simulink model "AreaCoverageTestHarness"  (R2016a)
settings: Solver=FixedStepDiscrete  StartTime=0.0  StopTime=16  FixedStep=0.005  RelTol=1e-3
undefined symbols (not defined in the file): EAST, ERRVAL, INIT_COMP_VALUE, INIT_X, INIT_Y, MAX_SPEED, NORTH, PLOT_SAMPLE, ROB_LENG, ROB_WHEEL_R, room, roomSize, SAMPLE_TIME, sigbuilder_block, SOUTH, STEP_SIZE, WEST
(part 1 of 2)
settings Model: Creator=oelkawok  LastModifiedBy=oelkawok

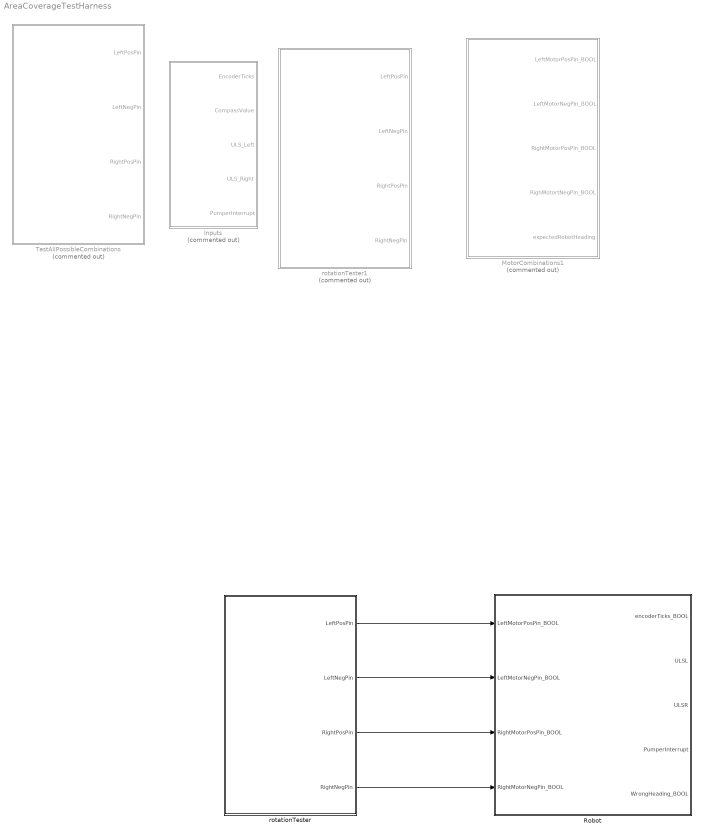
== system AreaCoverageTestHarness ==
  Inputs : Subsystem  Tag=STV Subsys  Commented=on  LoadFcn=sigbuilder_block('load');  StartFcn=sigbuilder_block('start');  StopFcn=sigbuilder_block('stop');  ClipboardFcn=sigbuilder_block('clipboard');  mask(Sigbuilder block){}
      mask help: Simulink:masks:SigbuilderBlock_MD
      mask init:
      | if ~strcmp(get_param(bdroot(gcbh),'SimulationStatus'),'stopped') tuvar = sigbuilder_block('maskInit'); end
      settings: CopyFcn=sigbuilder_block('copy');  DeleteFcn=sigbuilder_block('delete');  ModelCloseFcn=sigbuilder_block('modelClose');  PreSaveFcn=sigbuilder_block('preSave');  PauseFcn=sigbuilder_block('pause');  ContinueFcn=sigbuilder_block('continue');  NameChangeFcn=sigbuilder_block('namechange');  OpenFcn=sigbuilder_block('open',[211.2 103.8 550.8 400.2 ]);  CloseFcn=sigbuilder_block('close');
      mask Display: plot(0, 0, 100, 100,[2, 2, 32, 32, 2], [68, 8, 8, 68, 68],[32, 2], [38, 38], [32, 19, 2],[53, 60, 44], [32, 17, 17, 2],[16, 16, 31, 31]);txt = getActiveGroup(gcbh);text(2, 100, txt,'verticalAlignment', 'top');
  MotorCombinations1 : Subsystem  Commented=on
  Robot : Subsystem
  TestAllPossibleCombinations : Subsystem  Tag=STV Subsys  Commented=on  LoadFcn=sigbuilder_block('load');  StartFcn=sigbuilder_block('start');  StopFcn=sigbuilder_block('stop');  ClipboardFcn=sigbuilder_block('clipboard');  mask(Sigbuilder block){}
      mask help: Simulink:masks:SigbuilderBlock_MD
      mask init:
      | if ~strcmp(get_param(bdroot(gcbh),'SimulationStatus'),'stopped') tuvar = sigbuilder_block('maskInit'); end
      settings: CopyFcn=sigbuilder_block('copy');  DeleteFcn=sigbuilder_block('delete');  ModelCloseFcn=sigbuilder_block('modelClose');  PreSaveFcn=sigbuilder_block('preSave');  PauseFcn=sigbuilder_block('pause');  ContinueFcn=sigbuilder_block('continue');  NameChangeFcn=sigbuilder_block('namechange');  OpenFcn=sigbuilder_block('open',[5.4 28.8 1141.2 525 ]);  CloseFcn=sigbuilder_block('close');
      mask Display: plot(0, 0, 100, 100,[2, 2, 32, 32, 2], [68, 8, 8, 68, 68],[32, 2], [38, 38], [32, 19, 2],[53, 60, 44], [32, 17, 17, 2],[16, 16, 31, 31]);txt = getActiveGroup(gcbh);text(2, 100, txt,'verticalAlignment', 'top');
  rotationTester : Subsystem  Tag=STV Subsys  LoadFcn=sigbuilder_block('load',[6 28.2 1012.8 484.8 ]);  StartFcn=sigbuilder_block('start');  StopFcn=sigbuilder_block('stop');  ClipboardFcn=sigbuilder_block('clipboard');  mask(Sigbuilder block){}
      mask help: Simulink:masks:SigbuilderBlock_MD
      mask init:
      | if ~strcmp(get_param(bdroot(gcbh),'SimulationStatus'),'stopped') tuvar = sigbuilder_block('maskInit'); end
      settings: CopyFcn=sigbuilder_block('copy');  DeleteFcn=sigbuilder_block('delete');  ModelCloseFcn=sigbuilder_block('modelClose');  PreSaveFcn=sigbuilder_block('preSave');  PauseFcn=sigbuilder_block('pause');  ContinueFcn=sigbuilder_block('continue');  NameChangeFcn=sigbuilder_block('namechange');  OpenFcn=sigbuilder_block('open',[5.4 28.8 1141.2 525 ]);  CloseFcn=sigbuilder_block('close');
      mask Display: plot(0, 0, 100, 100,[2, 2, 32, 32, 2], [68, 8, 8, 68, 68],[32, 2], [38, 38], [32, 19, 2],[53, 60, 44], [32, 17, 17, 2],[16, 16, 31, 31]);txt = getActiveGroup(gcbh);text(2, 100, txt,'verticalAlignment', 'top');
  rotationTester1 : Subsystem  Tag=STV Subsys  Commented=on  LoadFcn=sigbuilder_block('load');  StartFcn=sigbuilder_block('start');  StopFcn=sigbuilder_block('stop');  ClipboardFcn=sigbuilder_block('clipboard');  mask(Sigbuilder block){}
      mask help: Simulink:masks:SigbuilderBlock_MD
      mask init:
      | if ~strcmp(get_param(bdroot(gcbh),'SimulationStatus'),'stopped') tuvar = sigbuilder_block('maskInit'); end
      settings: CopyFcn=sigbuilder_block('copy');  DeleteFcn=sigbuilder_block('delete');  ModelCloseFcn=sigbuilder_block('modelClose');  PreSaveFcn=sigbuilder_block('preSave');  PauseFcn=sigbuilder_block('pause');  ContinueFcn=sigbuilder_block('continue');  NameChangeFcn=sigbuilder_block('namechange');  OpenFcn=sigbuilder_block('open',[5.4 28.8 1141.2 525 ]);  CloseFcn=sigbuilder_block('close');
      mask Display: plot(0, 0, 100, 100,[2, 2, 32, 32, 2], [68, 8, 8, 68, 68],[32, 2], [38, 38], [32, 19, 2],[53, 60, 44], [32, 17, 17, 2],[16, 16, 31, 31]);txt = getActiveGroup(gcbh);text(2, 100, txt,'verticalAlignment', 'top');
  wires:
  rotationTester/1(LeftPosPin) -> Robot/1(LeftMotorPosPin_BOOL)
  rotationTester/2(LeftNegPin) -> Robot/2(LeftMotorNegPin_BOOL)
  rotationTester/4(RightNegPin) -> Robot/4(RightMotorNegPin_BOOL)
  rotationTester/3(RightPosPin) -> Robot/3(RightMotorPosPin_BOOL)

== system AreaCoverageTestHarness/Inputs ==
  Demux : Demux  Tag=STV Demux  Outputs=5
  FromWs : FromWorkspace  Tag=STV FromWs  VariableName=tuvar  SampleTime=0
      SigBuilderData=|
      | common.afterFinalStr = 'Extrapolate'
      | common.sampleTime = 0
      | dataSet.timeRange = [0 10]
      | dataSet.name = 'Group 1'
      | sbobj.Groups.Name = 'Group 1'
      | sbobj.Groups.Signals(1).Name = 'EncoderTicks'
      | sbobj.Groups.Signals(1).XData = [0 4 4 6 6 10]
      | sbobj.Groups.Signals(1).YData = [0 0 1 1 0 0]
      | sbobj.Groups.Signals(2).Name = 'CompassValue'
      | sbobj.Groups.Signals(2).XData = [0 4 4 6 6 10]
      | sbobj.Groups.Signals(2).YData = [0 0 1 1 0 0]
      | sbobj.Groups.Signals(3).Name = 'ULS_Left'
      | sbobj.Groups.Signals(3).XData = [0 4 4 6 6 10]
      | sbobj.Groups.Signals(3).YData = [0 0 1 1 0 0]
      | sbobj.Groups.Signals(4).Name = 'ULS_Right'
      | sbobj.Groups.Signals(4).XData = [0 4 4 6 6 10]
      | sbobj.Groups.Signals(4).YData = [0 0 1 1 0 0]
      | sbobj.Groups.Signals(5).Name = 'PumperInterrupt'
      | sbobj.Groups.Signals(5).XData = [0 4 4 6 6 10]
      | sbobj.Groups.Signals(5).YData = [0 0 1 1 0 0]
  EncoderTicks : Outport  Tag=STV Outport
  CompassValue : Outport  Tag=STV Outport  Port=2
  ULS_Left : Outport  Tag=STV Outport  Port=3
  ULS_Right : Outport  Tag=STV Outport  Port=4
  PumperInterrupt : Outport  Tag=STV Outport  Port=5
  wires:
  Demux/1 -> EncoderTicks/1
  FromWs/1 -> Demux/1
  Demux/2 -> CompassValue/1
  Demux/3 -> ULS_Left/1
  Demux/4 -> ULS_Right/1
  Demux/5 -> PumperInterrupt/1

== system AreaCoverageTestHarness/MotorCombinations1 ==
  Signal Builder : Subsystem  Tag=STV Subsys  LoadFcn=sigbuilder_block('load');  StartFcn=sigbuilder_block('start');  StopFcn=sigbuilder_block('stop');  ClipboardFcn=sigbuilder_block('clipboard');  mask(Sigbuilder block){}
      mask help: Simulink:masks:SigbuilderBlock_MD
      mask init:
      | if ~strcmp(get_param(bdroot(gcbh),'SimulationStatus'),'stopped') tuvar = sigbuilder_block('maskInit'); end
      settings: CopyFcn=sigbuilder_block('copy');  DeleteFcn=sigbuilder_block('delete');  ModelCloseFcn=sigbuilder_block('modelClose');  PreSaveFcn=sigbuilder_block('preSave');  PauseFcn=sigbuilder_block('pause');  ContinueFcn=sigbuilder_block('continue');  NameChangeFcn=sigbuilder_block('namechange');  OpenFcn=sigbuilder_block('open',[0 28.8 1152 564 ]);  CloseFcn=sigbuilder_block('close');
      mask Display: plot(0, 0, 100, 100,[2, 2, 32, 32, 2], [68, 8, 8, 68, 68],[32, 2], [38, 38], [32, 19, 2],[53, 60, 44], [32, 17, 17, 2],[16, 16, 31, 31]);txt = getActiveGroup(gcbh);text(2, 100, txt,'verticalAlignment', 'top');
  LeftMotorPosPin_BOOL : Outport
  LeftMotorNegPin_BOOL : Outport  Port=2
  RightMotorPosPin_BOOL : Outport  Port=3
  RighMotortNegPin_BOOL : Outport  Port=4
  expectedRobotHeading : Outport  Port=5
  wires:
  Signal Builder/5(expectedRobotHeading) -> expectedRobotHeading/1
  Signal Builder/1(LeftPosPin) -> LeftMotorPosPin_BOOL/1  "LeftMotorPosPin_BOOL"
  Signal Builder/2(LeftNegPin) -> LeftMotorNegPin_BOOL/1  "LeftMotorNegPin_BOOL"
  Signal Builder/3(RightPosPin) -> RightMotorPosPin_BOOL/1  "RightMotorPosPin_BOOL"
  Signal Builder/4(RightNegPin) -> RighMotortNegPin_BOOL/1  "RighMotortNegPin_BOOL"

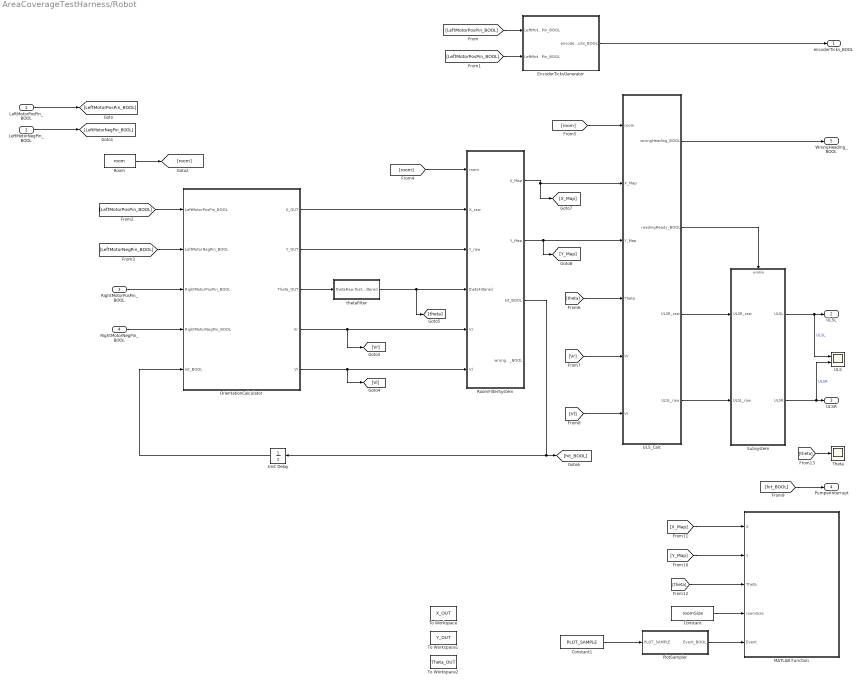
== system AreaCoverageTestHarness/Robot ==
  LeftMotorPosPin_BOOL : Inport
  LeftMotorNegPin_BOOL : Inport  Port=2
  RightMotorPosPin_BOOL : Inport  Port=3
  RightMotorNegPin_BOOL : Inport  Port=4
  Constant : Constant  Value=roomSize
  Constant1 : Constant  Value=PLOT_SAMPLE
  EncoderTicksGenerator : Subsystem
  MATLAB Function : MATLAB Function  TreatAsAtomicUnit=on
  OrientationCalculator : Subsystem
  PlotSampler : Stateflow chart  TreatAsAtomicUnit=on
  Room : Constant  Value=room
  RoomFilterSystem : Subsystem
  Subsystem : Subsystem
  Theta : Scope
  To Workspace : ToWorkspace  VariableName=X_OUT  SaveFormat=Timeseries  SampleTime=-1
  To Workspace1 : ToWorkspace  VariableName=Y_OUT  SaveFormat=Timeseries  SampleTime=-1
  To Workspace2 : ToWorkspace  VariableName=Theta_OUT  SaveFormat=Timeseries  SampleTime=-1
  ULS : Scope  NumInputPorts=2
  ULS_Calc : Subsystem
  Unit Delay : UnitDelay  SampleTime=-1
  thetaFilter : Subsystem
  encoderTicks_BOOL : Outport
  ULSL : Outport  Port=2
  ULSR : Outport  Port=3
  PumperInterrupt : Outport  Port=4
  WrongHeading_BOOL : Outport  Port=5
  wires:
  LeftMotorPosPin_BOOL/1 -> [LeftMotorPosPin_BOOL]
  LeftMotorNegPin_BOOL/1 -> [LeftMotorNegPin_BOOL]
  [LeftMotorPosPin_BOOL] -> EncoderTicksGenerator/2(LeftMotorNegPin_BOOL)
  [LeftMotorPosPin_BOOL] -> EncoderTicksGenerator/1(LeftMotorPosPin_BOOL)
  EncoderTicksGenerator/1(encoderTicks_BOOL) -> encoderTicks_BOOL/1
  [LeftMotorNegPin_BOOL] -> OrientationCalculator/2(LeftMotorNegPin_BOOL)
  [LeftMotorPosPin_BOOL] -> OrientationCalculator/1(LeftMotorPosPin_BOOL)
  RightMotorNegPin_BOOL/1 -> OrientationCalculator/4(RightMotorNegPin_BOOL)
  RightMotorPosPin_BOOL/1 -> OrientationCalculator/3(RightMotorPosPin_BOOL)
  OrientationCalculator/1(X_OUT) -> RoomFilterSystem/2(X_raw)
  OrientationCalculator/2(Y_OUT) -> RoomFilterSystem/3(Y_raw)
  OrientationCalculator/3(Theta_OUT) -> thetaFilter/1(thetaRaw)
  thetaFilter/1(thetaFiltered) -> RoomFilterSystem/4(thetaFiltered), [theta]
  OrientationCalculator/5(Vl) -> [Vl], RoomFilterSystem/6(Vl)
  OrientationCalculator/4(Vr) -> [Vr], RoomFilterSystem/5(Vr)
  RoomFilterSystem/3(hit_BOOL) -> [hit_BOOL], Unit Delay/1
  Unit Delay/1 -> OrientationCalculator/5(hit_BOOL)
  RoomFilterSystem/1(X_Map) -> [X_Map], ULS_Calc/2(X_Map)
  RoomFilterSystem/2(Y_Map) -> [Y_Map], ULS_Calc/3(Y_Map)
  Room/1 -> [room]
  [room] -> RoomFilterSystem/1(room)
  [room] -> ULS_Calc/1(room)
  [theta] -> ULS_Calc/4(Theta)
  [Vr] -> ULS_Calc/5(Vr)
  [Vl] -> ULS_Calc/6(Vl)
  ULS_Calc/2(readingReady_BOOL) -> Subsystem/Enable
  ULS_Calc/4(ULSL_raw) -> Subsystem/2(ULSL_raw)
  ULS_Calc/3(ULSR_raw) -> Subsystem/1(ULSR_raw)
  Subsystem/1(ULSL) -> ULS/1, ULSL/1  "ULSL"
  Subsystem/2(ULSR) -> ULS/2, ULSR/1  "ULSR"
  [hit_BOOL] -> PumperInterrupt/1
  ULS_Calc/1(wrongHeading_BOOL) -> WrongHeading_BOOL/1
  [theta] -> Theta/1
  [Y_Map] -> MATLAB Function/2(Y)
  [X_Map] -> MATLAB Function/1(X)
  [theta] -> MATLAB Function/3(Theta)
  Constant/1 -> MATLAB Function/4(roomSize)
  PlotSampler/1(Event_BOOL) -> MATLAB Function/5(Event)
  Constant1/1 -> PlotSampler/1(PLOT_SAMPLE)

== system AreaCoverageTestHarness/TestAllPossibleCombinations ==
  Demux : Demux  Tag=STV Demux
  FromWs : FromWorkspace  Tag=STV FromWs  VariableName=tuvar  SampleTime=0
      SigBuilderData=|
      | common.afterFinalStr = 'Extrapolate'
      | common.sampleTime = 0
      | dataSet.timeRange = [0 16]
      | dataSet.name = 'Group 1'
      | sbobj.Groups.Name = 'Group 1'
      | sbobj.Groups.Signals(1).Name = 'LeftPosPin'
      | sbobj.Groups.Signals(1).XData = [0 8 8 13.8 16]
      | sbobj.Groups.Signals(1).YData = [0 0 1 1 1]
      | sbobj.Groups.Signals(2).Name = 'LeftNegPin'
      | sbobj.Groups.Signals(2).XData = [0 1 2 4 4 8 8 12 12 16]
      | sbobj.Groups.Signals(2).YData = [0 0 0 0 1 1 0 0 1 1]
      | sbobj.Groups.Signals(3).Name = 'RightPosPin'
      | sbobj.Groups.Signals(3).XData = [0 1 2 4 4 6 8 8 10 10 12 12 14 14 16]
      | sbobj.Groups.Signals(3).YData = [0 0 0 0 1 1 1 0 0 1 1 0 0 1 1]
      | sbobj.Groups.Signals(4).Name = 'RightNegPin'
      | sbobj.Groups.Signals(4).XData = [0 1 1 3.08 3.08 8 11 11 12 12 13 13 14 14 15 15 16]
      | sbobj.Groups.Signals(4).YData = [0 0 1 1 0 0 0 1 1 0 0 1 1 0 0 1 1]
      | sbobj.Groups.TimeRange = [0 16]
  LeftPosPin : Outport  Tag=STV Outport
  LeftNegPin : Outport  Tag=STV Outport  Port=2
  RightPosPin : Outport  Tag=STV Outport  Port=3
  RightNegPin : Outport  Tag=STV Outport  Port=4
  wires:
  Demux/1 -> LeftPosPin/1
  FromWs/1 -> Demux/1
  Demux/2 -> LeftNegPin/1
  Demux/3 -> RightPosPin/1
  Demux/4 -> RightNegPin/1

== system AreaCoverageTestHarness/rotationTester ==
  Demux : Demux  Tag=STV Demux
  FromWs : FromWorkspace  Tag=STV FromWs  VariableName=tuvar  SampleTime=0
      SigBuilderData=|
      | common.afterFinalStr = 'Extrapolate'
      | common.sampleTime = 0
      | dataSet.timeRange = [0 16]
      | dataSet.name = 'Group 1'
      | sbobj.Groups.Name = 'Group 1'
      | sbobj.Groups.Signals(1).Name = 'LeftPosPin'
      | sbobj.Groups.Signals(1).XData = [0 2 3.35 8 8 12.16 12.16 16]
      | sbobj.Groups.Signals(1).YData = [1 1 1 1 0 0 1 1]
      | sbobj.Groups.Signals(2).Name = 'LeftNegPin'
      | sbobj.Groups.Signals(2).XData = [0 1 2.18 10 10 12 12 16]
      | sbobj.Groups.Signals(2).YData = [0 0 0 0 1 1 0 0]
      | sbobj.Groups.Signals(3).Name = 'RightPosPin'
      | sbobj.Groups.Signals(3).XData = [0 1 2 8 12.28 12.28 16]
      | sbobj.Groups.Signals(3).YData = [0 0 0 0 0 1 1]
      | sbobj.Groups.Signals(4).Name = 'RightNegPin'
      | sbobj.Groups.Signals(4).XData = [0 2 3.35 8 8 10 10 12 12 16]
      | sbobj.Groups.Signals(4).YData = [1 1 1 1 0 0 1 1 0 0]
      | sbobj.Groups.TimeRange = [0 16]
  LeftPosPin : Outport  Tag=STV Outport
  LeftNegPin : Outport  Tag=STV Outport  Port=2
  RightPosPin : Outport  Tag=STV Outport  Port=3
  RightNegPin : Outport  Tag=STV Outport  Port=4
  wires:
  Demux/4 -> RightNegPin/1
  Demux/3 -> RightPosPin/1
  Demux/2 -> LeftNegPin/1
  FromWs/1 -> Demux/1
  Demux/1 -> LeftPosPin/1

== system AreaCoverageTestHarness/rotationTester1 ==
  Demux : Demux  Tag=STV Demux
  FromWs : FromWorkspace  Tag=STV FromWs  VariableName=tuvar  SampleTime=0
      SigBuilderData=|
      | common.afterFinalStr = 'Extrapolate'
      | common.sampleTime = 0
      | dataSet.timeRange = [0 16]
      | dataSet.name = 'Group 1'
      | sbobj.Groups.Name = 'Group 1'
      | sbobj.Groups.Signals(1).Name = 'LeftPosPin'
      | sbobj.Groups.Signals(1).XData = [0 2.14 2.14 13.8 16]
      | sbobj.Groups.Signals(1).YData = [0 0 1 1 1]
      | sbobj.Groups.Signals(2).Name = 'LeftNegPin'
      | sbobj.Groups.Signals(2).XData = [0 1 1 2.08 2.08 12 16]
      | sbobj.Groups.Signals(2).YData = [0 0 1 1 0 0 0]
      | sbobj.Groups.Signals(3).Name = 'RightPosPin'
      | sbobj.Groups.Signals(3).XData = [0 1 2.08 2.08 13.18 14 14 16]
      | sbobj.Groups.Signals(3).YData = [0 0 0 1 1 1 0 0]
      | sbobj.Groups.Signals(4).Name = 'RightNegPin'
      | sbobj.Groups.Signals(4).XData = [0 1 1 8 11 12 13 14 15 16]
      | sbobj.Groups.Signals(4).YData = [0 0 1 1 1 1 1 1 1 1]
      | sbobj.Groups.TimeRange = [0 16]
  LeftPosPin : Outport  Tag=STV Outport
  LeftNegPin : Outport  Tag=STV Outport  Port=2
  RightPosPin : Outport  Tag=STV Outport  Port=3
  RightNegPin : Outport  Tag=STV Outport  Port=4
  wires:
  Demux/1 -> LeftPosPin/1
  FromWs/1 -> Demux/1
  Demux/2 -> LeftNegPin/1
  Demux/3 -> RightPosPin/1
  Demux/4 -> RightNegPin/1

== system AreaCoverageTestHarness/MotorCombinations1/Signal Builder ==
  Demux : Demux  Tag=STV Demux  Outputs=5
  FromWs : FromWorkspace  Tag=STV FromWs  VariableName=tuvar  SampleTime=0
      SigBuilderData=|
      | common.afterFinalStr = 'Extrapolate'
      | common.sampleTime = 0
      | dataSet.timeRange = [0 16]
      | dataSet.name = 'Group 1'
      | sbobj.Groups.Name = 'Group 1'
      | sbobj.Groups.Signals(1).Name = 'LeftPosPin'
      | sbobj.Groups.Signals(1).XData = [0 8 8 13.8 16]
      | sbobj.Groups.Signals(1).YData = [0 0 1 1 1]
      | sbobj.Groups.Signals(2).Name = 'LeftNegPin'
      | sbobj.Groups.Signals(2).XData = [0 1 2 4 4 8 8 12 12 16]
      | sbobj.Groups.Signals(2).YData = [0 0 0 0 1 1 0 0 1 1]
      | sbobj.Groups.Signals(3).Name = 'RightPosPin'
      | sbobj.Groups.Signals(3).XData = [0 1 2 2 4 4 6 6 8 8 10 10 12 12 14 14 16]
      | sbobj.Groups.Signals(3).YData = [0 0 0 1 1 0 0 1 1 0 0 1 1 0 0 1 1]
      | sbobj.Groups.Signals(4).Name = 'RightNegPin'
      | sbobj.Groups.Signals(4).XData = [0 1 1 2 2 3 3 4 4 5 5 6 6 7 7 8 8 9 9 10 10 11 11 12 12 13 13 14 14 15 15 16]
      | sbobj.Groups.Signals(4).YData = [0 0 1 1 0 0 1 1 0 0 1 1 0 0 1 1 0 0 1 1 0 0 1 1 0 0 1 1 0 0 1 1]
      | sbobj.Groups.Signals(5).Name = 'expectedRobotHeading'
      | sbobj.Groups.Signals(5).XData = [0 1 1 2 2 3 3 4 4 5 5 6 6 7 7 8 8 9 9 10 10 11 11 12 12 13 13 14 14 15 15 16]
      | sbobj.Groups.Signals(5).YData = [7 7 2 2 1 1 7 7 1 1 6 6 3 3 1 1 2 2 4 4 5 5 2 2 7 7 2 2 1 1 7 7]
      | sbobj.Groups.TimeRange = [0 16]
  LeftPosPin : Outport  Tag=STV Outport
  LeftNegPin : Outport  Tag=STV Outport  Port=2
  RightPosPin : Outport  Tag=STV Outport  Port=3
  RightNegPin : Outport  Tag=STV Outport  Port=4
  expectedRobotHeading : Outport  Tag=STV Outport  Port=5
  wires:
  Demux/5 -> expectedRobotHeading/1
  Demux/4 -> RightNegPin/1
  Demux/3 -> RightPosPin/1
  Demux/2 -> LeftNegPin/1
  FromWs/1 -> Demux/1
  Demux/1 -> LeftPosPin/1

== system AreaCoverageTestHarness/Robot/EncoderTicksGenerator ==
  LeftMotorPosPin_BOOL : Inport
  LeftMotorNegPin_BOOL : Inport  Port=2
  Logical Operator : Logic  Operator=XOR  AllPortsSameDT=off  OutDataTypeStr=boolean
  SquareWaveCreatorLeft : Stateflow chart  TreatAsAtomicUnit=on
  encoderTicks_BOOL : Outport
  wires:
  LeftMotorNegPin_BOOL/1 -> Logical Operator/2
  LeftMotorPosPin_BOOL/1 -> Logical Operator/1
  Logical Operator/1 -> SquareWaveCreatorLeft/1(ControlSignal_BOOL_in)
  SquareWaveCreatorLeft/1(encoderTicks_BOOL) -> encoderTicks_BOOL/1

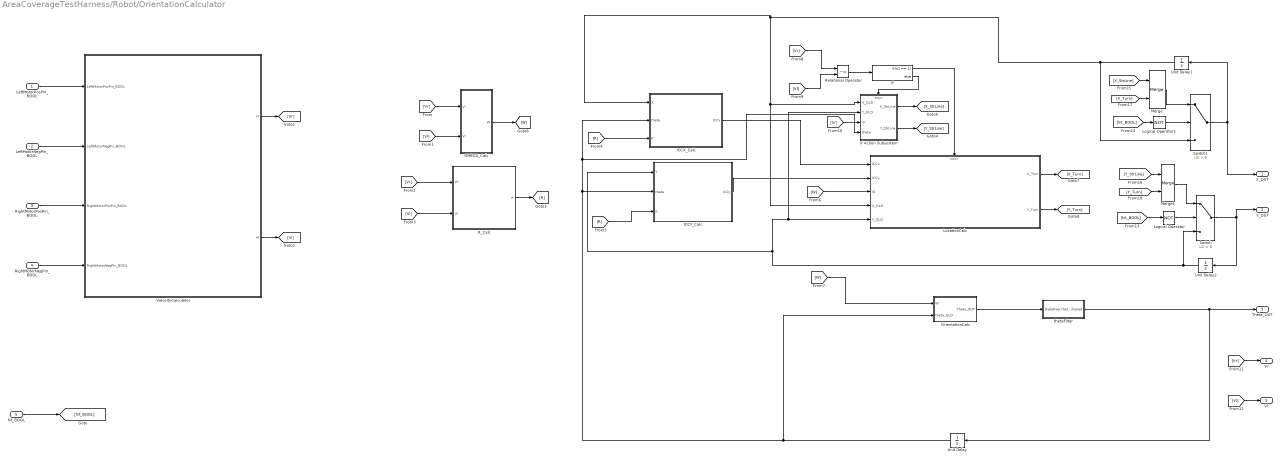
== system AreaCoverageTestHarness/Robot/OrientationCalculator ==
  LeftMotorPosPin_BOOL : Inport
  LeftMotorNegPin_BOOL : Inport  Port=2
  RightMotorPosPin_BOOL : Inport  Port=3
  RightMotorNegPin_BOOL : Inport  Port=4
  hit_BOOL : Inport  Port=5
  ICCX_Calc : Subsystem
  ICCY_Calc : Subsystem
  If : If  IfExpression=u1 == 1
  If Action Subsystem : Subsystem  TreatAsAtomicUnit=on
  LocationCalc : Subsystem
  Logical Operator : Logic  Operator=NOT  AllPortsSameDT=off  OutDataTypeStr=boolean
  Logical Operator1 : Logic  Operator=NOT  AllPortsSameDT=off  OutDataTypeStr=boolean
  Merge : Merge
  Merge1 : Merge
  OMEGA_Calc : Subsystem
  OrientationCalc : Subsystem
  R_Calc : Subsystem
  Relational Operator : RelationalOperator  Operator=~=  OutDataTypeStr=boolean
  Switch : Switch  Criteria=u2 > Threshold
  Switch1 : Switch  Criteria=u2 > Threshold
  Unit Delay : UnitDelay  InitialCondition=INIT_COMP_VALUE  SampleTime=-1
  Unit Delay1 : UnitDelay  InitialCondition=INIT_X  SampleTime=-1
  Unit Delay2 : UnitDelay  InitialCondition=INIT_Y  SampleTime=-1
  VelocityCalculator : Subsystem
  thetaFilter : Subsystem
  X_OUT : Outport
  Y_OUT : Outport  Port=2
  Theta_OUT : Outport  Port=3
  Vr : Outport  Port=4
  Vl : Outport  Port=5
  wires:
  [Vr] -> OMEGA_Calc/1(Vr)
  [Vl] -> OMEGA_Calc/2(Vl)
  [Vr] -> R_Calc/1(Vr)
  [Vl] -> R_Calc/2(Vl)
  R_Calc/1(R) -> [R]
  Unit Delay1/1 -> ICCX_Calc/1(X), If Action Subsystem/1(X_OLD), LocationCalc/4(X_OLD), Switch1/3
  Unit Delay/1 -> OrientationCalc/2(theta_OLD), ICCY_Calc/2(theta), If Action Subsystem/4(theta), ICCX_Calc/2(theta)
  [R] -> ICCX_Calc/3(R)
  Unit Delay2/1 -> Switch/3, ICCY_Calc/1(Y), If Action Subsystem/2(Y_OLD), LocationCalc/5(Y_OLD)
  [R] -> ICCY_Calc/3(R)
  ICCX_Calc/1(ICCx) -> LocationCalc/1(ICCx)
  ICCY_Calc/1(ICCy) -> LocationCalc/2(ICCy)
  OMEGA_Calc/1(W) -> [W]
  Merge1/1 -> Switch/1
  [W] -> LocationCalc/3(W)
  OrientationCalc/1(Theta_OUT) -> thetaFilter/1(thetaRaw)
  [W] -> OrientationCalc/1(W)
  [Vl] -> Relational Operator/2
  [Vr] -> Relational Operator/1
  Relational Operator/1 -> If/1
  If/1 -> LocationCalc/Action
  If/2 -> If Action Subsystem/Action
  [Vr] -> If Action Subsystem/3(Vr)
  thetaFilter/1(thetaFiltered) -> Unit Delay/1, Theta_OUT/1
  [Vl] -> Vl/1
  [Vr] -> Vr/1
  hit_BOOL/1 -> [hit_BOOL]
  [hit_BOOL] -> Logical Operator/1
  Logical Operator/1 -> Switch/2
  Switch/1 -> Unit Delay2/1, Y_OUT/1
  [hit_BOOL] -> Logical Operator1/1
  Logical Operator1/1 -> Switch1/2
  Merge/1 -> Switch1/1
  Switch1/1 -> Unit Delay1/1, X_OUT/1
  LeftMotorPosPin_BOOL/1 -> VelocityCalculator/1(LeftMotorPosPin_BOOL)
  LeftMotorNegPin_BOOL/1 -> VelocityCalculator/2(LeftMotorNegPin_BOOL)
  RightMotorPosPin_BOOL/1 -> VelocityCalculator/3(RightMotorPosPin_BOOL)
  RightMotorNegPin_BOOL/1 -> VelocityCalculator/4(RightMotorNegPin_BOOL)
  VelocityCalculator/1(Vr) -> [Vr]
  VelocityCalculator/2(Vl) -> [Vl]
  [X_StrLine] -> Merge/1
  If Action Subsystem/1(X_StrLine) -> [X_StrLine]
  If Action Subsystem/2(Y_StrLine) -> [Y_StrLine]
  [Y_StrLine] -> Merge1/1
  LocationCalc/1(X_Turn) -> [X_Turn]
  [X_Turn] -> Merge/2
  LocationCalc/2(Y_Turn) -> [Y_Turn]
  [Y_Turn] -> Merge1/2

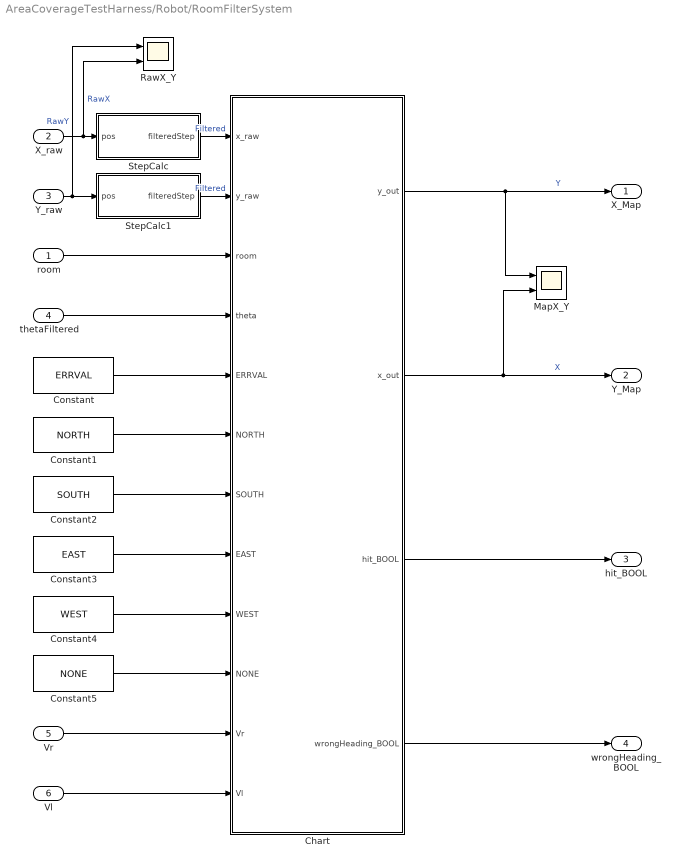
== system AreaCoverageTestHarness/Robot/RoomFilterSystem ==
  room : Inport
  X_raw : Inport  Port=2
  Y_raw : Inport  Port=3
  thetaFiltered : Inport  Port=4
  Vr : Inport  Port=5
  Vl : Inport  Port=6
  Chart : Stateflow chart  TreatAsAtomicUnit=on
  Constant : Constant  Value=ERRVAL
  Constant1 : Constant  Value=NORTH
  Constant2 : Constant  Value=SOUTH
  Constant3 : Constant  Value=EAST
  Constant4 : Constant  Value=WEST
  Constant5 : Constant  Value=NONE
  MapX_Y : Scope  NumInputPorts=2
  RawX_Y : Scope  NumInputPorts=2
  StepCalc : Subsystem
  StepCalc1 : Subsystem
  X_Map : Outport
  Y_Map : Outport  Port=2
  hit_BOOL : Outport  Port=3
  wrongHeading_BOOL : Outport  Port=4
  wires:
  Y_raw/1 -> RawX_Y/1, StepCalc1/1(pos)  "RawY"
  room/1 -> Chart/3(room)
  Chart/1(y_out) -> MapX_Y/1, X_Map/1  "Y"
  Chart/2(x_out) -> MapX_Y/2, Y_Map/1  "X"
  thetaFiltered/1 -> Chart/4(theta)
  Constant/1 -> Chart/5(ERRVAL)
  Constant1/1 -> Chart/6(NORTH)
  Constant2/1 -> Chart/7(SOUTH)
  Constant5/1 -> Chart/10(NONE)
  Constant4/1 -> Chart/9(WEST)
  Constant3/1 -> Chart/8(EAST)
  Vr/1 -> Chart/11(Vr)
  Vl/1 -> Chart/12(Vl)
  Chart/3(hit_BOOL) -> hit_BOOL/1
  Chart/4(wrongHeading_BOOL) -> wrongHeading_BOOL/1
  StepCalc1/1(filteredStep) -> Chart/2(y_raw)  "Filtered"
  X_raw/1 -> RawX_Y/2, StepCalc/1(pos)  "RawX"
  StepCalc/1(filteredStep) -> Chart/1(x_raw)  "Filtered"

== system AreaCoverageTestHarness/Robot/Subsystem ==
  ULSR_raw : Inport
  ULSL_raw : Inport  Port=2
  Enable : EnablePort
  ULSL : Outport
  ULSR : Outport  Port=2
  wires:
  ULSL_raw/1 -> ULSR/1
  ULSR_raw/1 -> ULSL/1

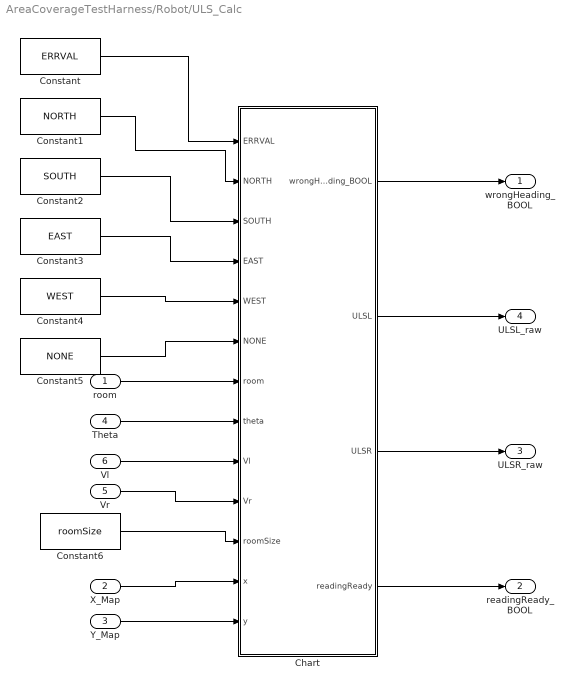
== system AreaCoverageTestHarness/Robot/ULS_Calc ==
  room : Inport
  X_Map : Inport  Port=2
  Y_Map : Inport  Port=3
  Theta : Inport  Port=4
  Vr : Inport  Port=5
  Vl : Inport  Port=6
  Chart : Stateflow chart  TreatAsAtomicUnit=on
  Constant : Constant  Value=ERRVAL
  Constant1 : Constant  Value=NORTH
  Constant2 : Constant  Value=SOUTH
  Constant3 : Constant  Value=EAST
  Constant4 : Constant  Value=WEST
  Constant5 : Constant  Value=NONE
  Constant6 : Constant  Value=roomSize
  wrongHeading_BOOL : Outport
  readingReady_BOOL : Outport  Port=2
  ULSR_raw : Outport  Port=3
  ULSL_raw : Outport  Port=4
  wires:
  X_Map/1 -> Chart/12(x)
  Y_Map/1 -> Chart/13(y)
  Theta/1 -> Chart/8(theta)
  Constant4/1 -> Chart/5(WEST)
  Constant5/1 -> Chart/6(NONE)
  Constant3/1 -> Chart/4(EAST)
  Constant2/1 -> Chart/3(SOUTH)
  Constant1/1 -> Chart/2(NORTH)
  Constant/1 -> Chart/1(ERRVAL)
  room/1 -> Chart/7(room)
  Constant6/1 -> Chart/11(roomSize)
  Vl/1 -> Chart/9(Vl)
  Vr/1 -> Chart/10(Vr)
  Chart/2(ULSL) -> ULSL_raw/1
  Chart/3(ULSR) -> ULSR_raw/1
  Chart/4(readingReady) -> readingReady_BOOL/1
  Chart/1(wrongHeading_BOOL) -> wrongHeading_BOOL/1

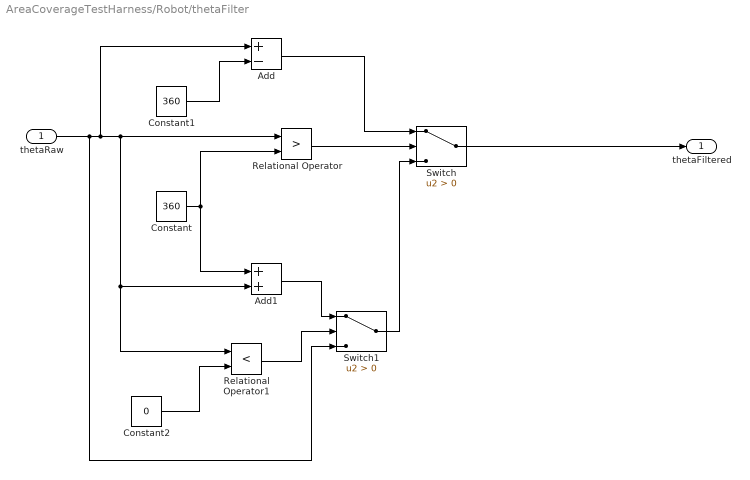
== system AreaCoverageTestHarness/Robot/thetaFilter ==
  thetaRaw : Inport
  Add : Sum  Inputs=+-
  Add1 : Sum
  Constant : Constant  Value=360
  Constant1 : Constant  Value=360
  Constant2 : Constant  Value=0
  Relational Operator : RelationalOperator  Operator=>  OutDataTypeStr=boolean
  Relational Operator1 : RelationalOperator  Operator=<  OutDataTypeStr=boolean
  Switch : Switch  Criteria=u2 > Threshold
  Switch1 : Switch  Criteria=u2 > Threshold
  thetaFiltered : Outport
  wires:
  thetaRaw/1 -> Switch1/3, Add/1, Add1/2, Relational Operator1/1, Relational Operator/1
  Constant/1 -> Add1/1, Relational Operator/2
  Relational Operator/1 -> Switch/2
  Constant1/1 -> Add/2
  Add/1 -> Switch/1
  Constant2/1 -> Relational Operator1/2
  Relational Operator1/1 -> Switch1/2
  Add1/1 -> Switch1/1
  Switch1/1 -> Switch/3
  Switch/1 -> thetaFiltered/1

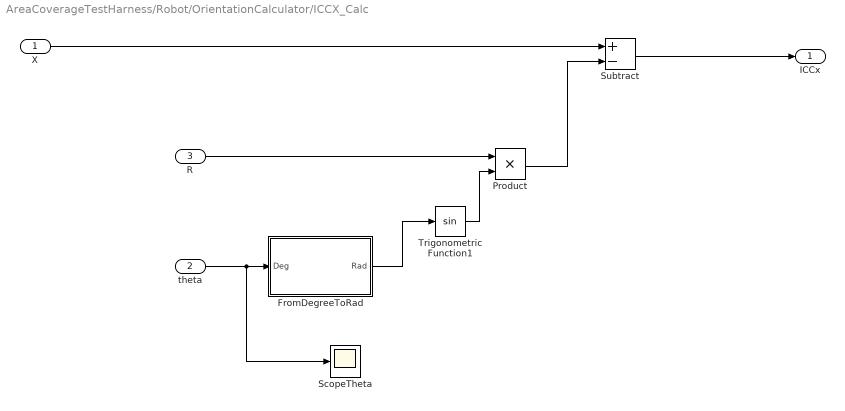
== system AreaCoverageTestHarness/Robot/OrientationCalculator/ICCX_Calc ==
  X : Inport
  theta : Inport  Port=2
  R : Inport  Port=3
  FromDegreeToRad : Subsystem
  Product : Product
  ScopeTheta : Scope
  Subtract : Sum  Inputs=+-
  Trigonometric Function1 : Trigonometry
  ICCx : Outport
  wires:
  Product/1 -> Subtract/2
  X/1 -> Subtract/1
  FromDegreeToRad/1(Rad) -> Trigonometric Function1/1
  Subtract/1 -> ICCx/1
  theta/1 -> ScopeTheta/1, FromDegreeToRad/1(Deg)
  Trigonometric Function1/1 -> Product/2
  R/1 -> Product/1

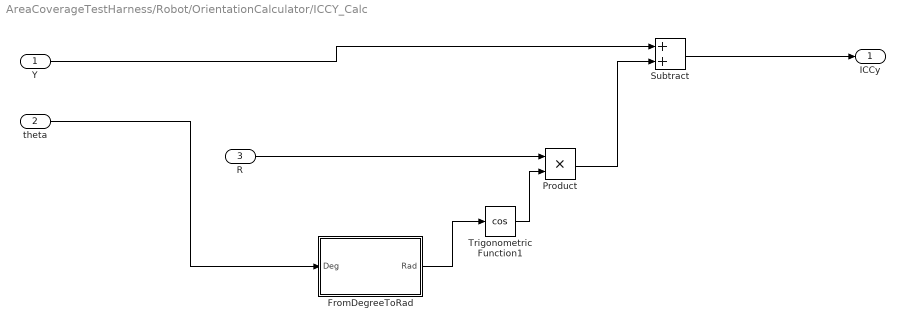
== system AreaCoverageTestHarness/Robot/OrientationCalculator/ICCY_Calc ==
  Y : Inport
  theta : Inport  Port=2
  R : Inport  Port=3
  FromDegreeToRad : Subsystem
  Product : Product
  Subtract : Sum
  Trigonometric Function1 : Trigonometry  Operator=cos
  ICCy : Outport
  wires:
  Y/1 -> Subtract/1
  Trigonometric Function1/1 -> Product/2
  theta/1 -> FromDegreeToRad/1(Deg)
  Subtract/1 -> ICCy/1
  FromDegreeToRad/1(Rad) -> Trigonometric Function1/1
  Product/1 -> Subtract/2
  R/1 -> Product/1

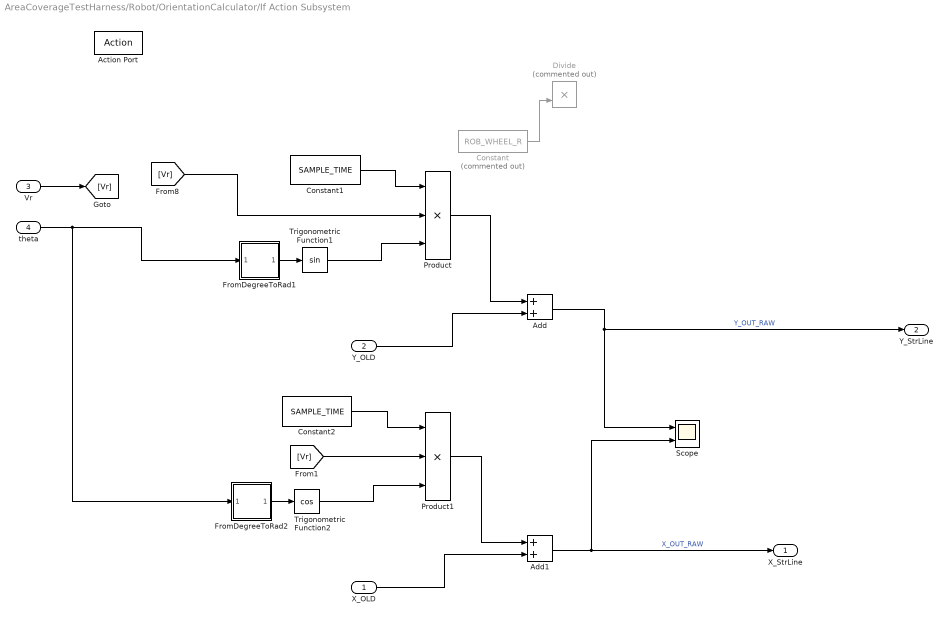
== system AreaCoverageTestHarness/Robot/OrientationCalculator/If Action Subsystem ==
  X_OLD : Inport
  Y_OLD : Inport  Port=2
  Vr : Inport  Port=3
  theta : Inport  Port=4
  Action Port : ActionPort  ActionType=else
  Add : Sum
  Add1 : Sum
  Constant : Constant  Commented=on  Value=ROB_WHEEL_R
  Constant1 : Constant  Value=SAMPLE_TIME  SampleTime=-1
  Constant2 : Constant  Value=SAMPLE_TIME  SampleTime=-1
  Divide : Product  Commented=on  Inputs=**
  FromDegreeToRad1 : Subsystem
  FromDegreeToRad2 : Subsystem
  Product : Product  Inputs=3
  Product1 : Product  Inputs=3
  Scope : Scope  NumInputPorts=2
  Trigonometric Function1 : Trigonometry
  Trigonometric Function2 : Trigonometry  Operator=cos
  X_StrLine : Outport
  Y_StrLine : Outport  Port=2
  wires:
  FromDegreeToRad1/1(Rad) -> Trigonometric Function1/1
  Trigonometric Function1/1 -> Product/3
  Vr/1 -> [Vr]
  theta/1 -> FromDegreeToRad2/1(Deg), FromDegreeToRad1/1(Deg)
  Constant1/1 -> Product/1
  Y_OLD/1 -> Add/2
  Product/1 -> Add/1
  Add/1 -> Y_StrLine/1, Scope/1  "Y_OUT_RAW"
  FromDegreeToRad2/1(Rad) -> Trigonometric Function2/1
  Trigonometric Function2/1 -> Product1/3
  [Vr] -> Product1/2
  Constant2/1 -> Product1/1
  X_OLD/1 -> Add1/2
  Product1/1 -> Add1/1
  Add1/1 -> Scope/2, X_StrLine/1  "X_OUT_RAW"
  [Vr] -> Product/2
  Constant/1 -> Divide/2

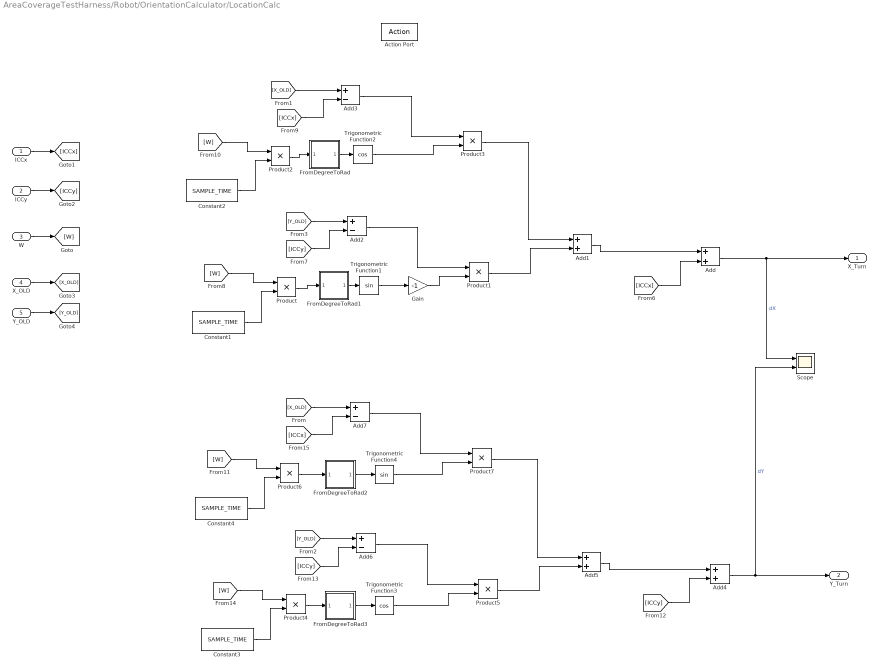
== system AreaCoverageTestHarness/Robot/OrientationCalculator/LocationCalc ==
  ICCx : Inport
  ICCy : Inport  Port=2
  W : Inport  Port=3
  X_OLD : Inport  Port=4
  Y_OLD : Inport  Port=5
  Action Port : ActionPort  ActionType=then
  Add{,1,4..5} (4 alike) : Sum
  Add{2..3,6..7} (4 alike) : Sum  Inputs=+-
  Constant{1..4} (4 alike) : Constant  Value=SAMPLE_TIME  SampleTime=-1
  FromDegreeToRad : Subsystem
  FromDegreeToRad1 : Subsystem
  FromDegreeToRad2 : Subsystem
  FromDegreeToRad3 : Subsystem
  Gain : Gain  Gain=-1
  Product{,1..7} (8 alike) : Product
  Scope : Scope  NumInputPorts=2
  Trigonometric Function1 : Trigonometry
  Trigonometric Function2 : Trigonometry  Operator=cos
  Trigonometric Function3 : Trigonometry  Operator=cos
  Trigonometric Function4 : Trigonometry
  X_Turn : Outport
  Y_Turn : Outport  Port=2
  wires:
  [W] -> Product/1
  Gain/1 -> Product1/2
  [ICCx] -> Add/2
  Add2/1 -> Product1/1
  Add1/1 -> Add/1
  Product2/1 -> FromDegreeToRad/1(Deg)
  Product1/1 -> Add1/2
  Constant1/1 -> Product/2
  Add3/1 -> Product3/1
  Add/1 -> Scope/1, X_Turn/1  "dX"
  Product/1 -> FromDegreeToRad1/1(Deg)
  Trigonometric Function1/1 -> Gain/1
  [ICCy] -> Add2/2
  Constant2/1 -> Product2/2
  Trigonometric Function2/1 -> Product3/2
  [ICCx] -> Add3/2
  [W] -> Product2/1
  Product3/1 -> Add1/1
  Add6/1 -> Product5/1
  [ICCy] -> Add4/2
  Product5/1 -> Add5/2
  Product7/1 -> Add5/1
  Add7/1 -> Product7/1
  Product6/1 -> FromDegreeToRad2/1(Deg)
  Trigonometric Function3/1 -> Product5/2
  Add5/1 -> Add4/1
  Trigonometric Function4/1 -> Product7/2
  [W] -> Product4/1
  Add4/1 -> Scope/2, Y_Turn/1  "dY"
  [ICCy] -> Add6/2
  [ICCx] -> Add7/2
  Constant3/1 -> Product4/2
  Product4/1 -> FromDegreeToRad3/1(Deg)
  [W] -> Product6/1
  Constant4/1 -> Product6/2
  W/1 -> [W]
  ICCx/1 -> [ICCx]
  ICCy/1 -> [ICCy]
  FromDegreeToRad/1(Rad) -> Trigonometric Function2/1
  FromDegreeToRad1/1(Rad) -> Trigonometric Function1/1
  FromDegreeToRad2/1(Rad) -> Trigonometric Function4/1
  FromDegreeToRad3/1(Rad) -> Trigonometric Function3/1
  X_OLD/1 -> [X_OLD]
  [X_OLD] -> Add7/1
  [X_OLD] -> Add3/1
  Y_OLD/1 -> [Y_OLD]
  [Y_OLD] -> Add6/1
  [Y_OLD] -> Add2/1

== system AreaCoverageTestHarness/Robot/OrientationCalculator/OMEGA_Calc ==
  Vr : Inport
  Vl : Inport  Port=2
  Add : Sum  Inputs=+-
  Constant3 : Constant  Value=ROB_LENG  OutDataTypeStr=int16
  Divide1 : Product  Inputs=*/
  W : Outport
  wires:
  Vl/1 -> Add/2
  Vr/1 -> Add/1
  Constant3/1 -> Divide1/2
  Divide1/1 -> W/1
  Add/1 -> Divide1/1

== system AreaCoverageTestHarness/Robot/OrientationCalculator/OrientationCalc ==
  W : Inport
  theta_OLD : Inport  Port=2
  Add : Sum
  Constant4 : Constant  Value=SAMPLE_TIME  SampleTime=-1
  Product : Product
  Theta_OUT : Outport
  wires:
  theta_OLD/1 -> Add/2
  Constant4/1 -> Product/2
  W/1 -> Product/1
  Add/1 -> Theta_OUT/1
  Product/1 -> Add/1

== system AreaCoverageTestHarness/Robot/OrientationCalculator/R_Calc ==
  Vr : Inport
  Vl : Inport  Port=2
  If : If  NumInputs=2  IfExpression=u1 ~= u2  ShowElse=off
  If Action Subsystem1 : Subsystem  TreatAsAtomicUnit=on
  R : Outport
  wires:
  If/1 -> If Action Subsystem1/Action
  If Action Subsystem1/1(R) -> R/1
  Vr/1 -> If/1, If Action Subsystem1/1(Vr)
  Vl/1 -> If/2, If Action Subsystem1/2(Vl)

== system AreaCoverageTestHarness/Robot/OrientationCalculator/VelocityCalculator ==
  LeftMotorPosPin_BOOL : Inport
  LeftMotorNegPin_BOOL : Inport  Port=2
  RightMotorPosPin_BOOL : Inport  Port=3
  RightMotorNegPin_BOOL : Inport  Port=4
  CCW_FAST : Constant  Value=MAX_SPEED  OutDataTypeStr=int16  SampleTime=-1
  Chart : Stateflow chart  TreatAsAtomicUnit=on
  Vr : Outport
  Vl : Outport  Port=2
  wires:
  LeftMotorNegPin_BOOL/1 -> Chart/2(LeftMotorNegPin_BOOL)
  RightMotorNegPin_BOOL/1 -> Chart/4(RightMotorNegPin_BOOL)
  LeftMotorPosPin_BOOL/1 -> Chart/1(LeftMotorPosPin_BOOL)
  CCW_FAST/1 -> Chart/5(MAX_SPEED)
  RightMotorPosPin_BOOL/1 -> Chart/3(RightMotorPosPin_BOOL)
  Chart/1(Vr) -> Vr/1
  Chart/2(Vl) -> Vl/1

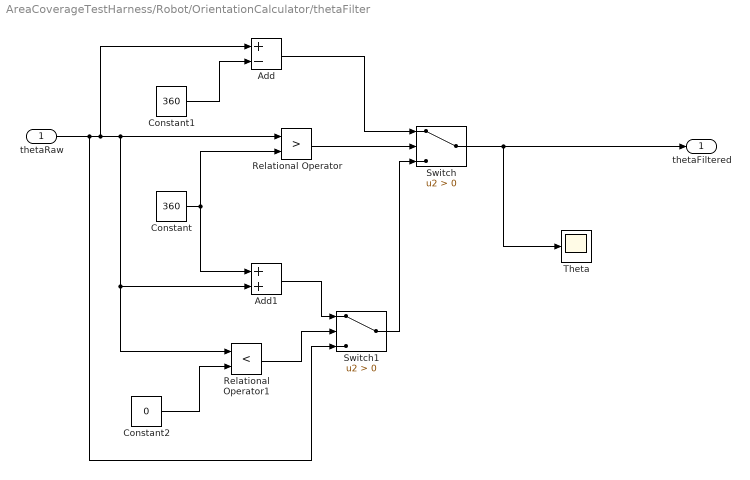
== system AreaCoverageTestHarness/Robot/OrientationCalculator/thetaFilter ==
  thetaRaw : Inport
  Add : Sum  Inputs=+-
  Add1 : Sum
  Constant : Constant  Value=360
  Constant1 : Constant  Value=360
  Constant2 : Constant  Value=0
  Relational Operator : RelationalOperator  Operator=>  OutDataTypeStr=boolean
  Relational Operator1 : RelationalOperator  Operator=<  OutDataTypeStr=boolean
  Switch : Switch  Criteria=u2 > Threshold
  Switch1 : Switch  Criteria=u2 > Threshold
  Theta : Scope
  thetaFiltered : Outport
  wires:
  thetaRaw/1 -> Switch1/3, Add/1, Add1/2, Relational Operator1/1, Relational Operator/1
  Constant/1 -> Add1/1, Relational Operator/2
  Relational Operator/1 -> Switch/2
  Constant1/1 -> Add/2
  Add/1 -> Switch/1
  Constant2/1 -> Relational Operator1/2
  Relational Operator1/1 -> Switch1/2
  Add1/1 -> Switch1/1
  Switch1/1 -> Switch/3
  Switch/1 -> Theta/1, thetaFiltered/1

== system AreaCoverageTestHarness/Robot/RoomFilterSystem/StepCalc ==
  pos : Inport
  Chart : Stateflow chart  TreatAsAtomicUnit=on
  Data Type Conversion : DataTypeConversion  OutDataTypeStr=int32
  STEP_SIZE : Constant  Value=STEP_SIZE  OutDataTypeStr=int8
  Unit Delay : UnitDelay  SampleTime=-1
  filteredStep : Outport
  wires:
  pos/1 -> Data Type Conversion/1
  Unit Delay/1 -> Chart/2(oldPos)
  Chart/1(step) -> filteredStep/1
  Data Type Conversion/1 -> Chart/1(pos), Unit Delay/1
  STEP_SIZE/1 -> Chart/3(STEP_SIZE)

== system AreaCoverageTestHarness/Robot/RoomFilterSystem/StepCalc1 ==
  pos : Inport
  Chart : Stateflow chart  TreatAsAtomicUnit=on
  Data Type Conversion : DataTypeConversion  OutDataTypeStr=int32
  STEP_SIZE : Constant  Value=STEP_SIZE  OutDataTypeStr=int8
  Unit Delay : UnitDelay  SampleTime=-1
  filteredStep : Outport
  wires:
  STEP_SIZE/1 -> Chart/3(STEP_SIZE)
  Data Type Conversion/1 -> Unit Delay/1, Chart/1(pos)
  Chart/1(step) -> filteredStep/1
  Unit Delay/1 -> Chart/2(oldPos)
  pos/1 -> Data Type Conversion/1

== system AreaCoverageTestHarness/Robot/OrientationCalculator/ICCX_Calc/FromDegreeToRad ==
  Deg : Inport
  Constant1 : Constant  Value=pi
  Constant2 : Constant  Value=180
  Divide : Product  Inputs=*/
  Product : Product
  Rad : Outport
  wires:
  Divide/1 -> Product/1
  Deg/1 -> Product/2
  Constant1/1 -> Divide/1
  Product/1 -> Rad/1
  Constant2/1 -> Divide/2

== system AreaCoverageTestHarness/Robot/OrientationCalculator/ICCY_Calc/FromDegreeToRad ==
  Deg : Inport
  Constant1 : Constant  Value=pi
  Constant2 : Constant  Value=180
  Divide : Product  Inputs=*/
  Product : Product
  Rad : Outport
  wires:
  Divide/1 -> Product/1
  Deg/1 -> Product/2
  Constant1/1 -> Divide/1
  Product/1 -> Rad/1
  Constant2/1 -> Divide/2

== system AreaCoverageTestHarness/Robot/OrientationCalculator/If Action Subsystem/FromDegreeToRad1 ==
  Deg : Inport
  Constant1 : Constant  Value=pi
  Constant2 : Constant  Value=180
  Divide : Product  Inputs=*/
  Product : Product
  Rad : Outport
  wires:
  Constant2/1 -> Divide/2
  Product/1 -> Rad/1
  Constant1/1 -> Divide/1
  Deg/1 -> Product/2
  Divide/1 -> Product/1

== system AreaCoverageTestHarness/Robot/OrientationCalculator/If Action Subsystem/FromDegreeToRad2 ==
  Deg : Inport
  Constant1 : Constant  Value=pi
  Constant2 : Constant  Value=180
  Divide : Product  Inputs=*/
  Product : Product
  Rad : Outport
  wires:
  Divide/1 -> Product/1
  Deg/1 -> Product/2
  Constant1/1 -> Divide/1
  Product/1 -> Rad/1
  Constant2/1 -> Divide/2

== system AreaCoverageTestHarness/Robot/OrientationCalculator/LocationCalc/FromDegreeToRad ==
  Deg : Inport
  Constant1 : Constant  Value=pi
  Constant2 : Constant  Value=180
  Divide : Product  Inputs=*/
  Product : Product
  Rad : Outport
  wires:
  Divide/1 -> Product/1
  Deg/1 -> Product/2
  Constant1/1 -> Divide/1
  Product/1 -> Rad/1
  Constant2/1 -> Divide/2

== system AreaCoverageTestHarness/Robot/OrientationCalculator/LocationCalc/FromDegreeToRad1 ==
  Deg : Inport
  Constant1 : Constant  Value=pi
  Constant2 : Constant  Value=180
  Divide : Product  Inputs=*/
  Product : Product
  Rad : Outport
  wires:
  Constant2/1 -> Divide/2
  Product/1 -> Rad/1
  Constant1/1 -> Divide/1
  Deg/1 -> Product/2
  Divide/1 -> Product/1

== system AreaCoverageTestHarness/Robot/OrientationCalculator/LocationCalc/FromDegreeToRad2 ==
  Deg : Inport
  Constant1 : Constant  Value=pi
  Constant2 : Constant  Value=180
  Divide : Product  Inputs=*/
  Product : Product
  Rad : Outport
  wires:
  Divide/1 -> Product/1
  Deg/1 -> Product/2
  Constant1/1 -> Divide/1
  Product/1 -> Rad/1
  Constant2/1 -> Divide/2

== system AreaCoverageTestHarness/Robot/OrientationCalculator/LocationCalc/FromDegreeToRad3 ==
  Deg : Inport
  Constant1 : Constant  Value=pi
  Constant2 : Constant  Value=180
  Divide : Product  Inputs=*/
  Product : Product
  Rad : Outport
  wires:
  Constant2/1 -> Divide/2
  Product/1 -> Rad/1
  Constant1/1 -> Divide/1
  Deg/1 -> Product/2
  Divide/1 -> Product/1

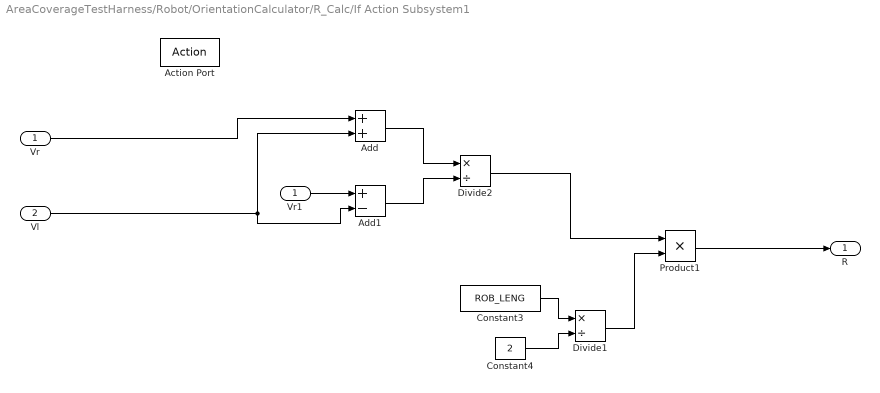
== system AreaCoverageTestHarness/Robot/OrientationCalculator/R_Calc/If Action Subsystem1 ==
  Vr : Inport
  Vl : Inport  Port=2
  Action Port : ActionPort  ActionType=then
  Add : Sum
  Add1 : Sum  Inputs=+-
  Constant3 : Constant  Value=ROB_LENG
  Constant4 : Constant  Value=2  OutDataTypeStr=int16
  Divide1 : Product  Inputs=*/
  Divide2 : Product  Inputs=*/
  Product1 : Product
  Vr1 : InportShadow
  R : Outport  OutputWhenDisabled=reset  InitialOutput=0
      settings: AttributesFormatString=%<OutputWhenDisabled>
  wires:
  Vr1/1 -> Add1/1
  Vr/1 -> Add/1
  Add1/1 -> Divide2/2
  Add/1 -> Divide2/1
  Divide1/1 -> Product1/2
  Divide2/1 -> Product1/1
  Constant3/1 -> Divide1/1
  Product1/1 -> R/1
  Vl/1 -> Add1/2, Add/2
  Constant4/1 -> Divide1/2

== stateflow chart AreaCoverageTestHarness/Robot/RoomFilterSystem/Chart ==
  state noHit
    entry:
    hit_BOOL = false;
  state HitCalcHeading
    entry:
    hit_BOOL = true;
    during:
    c_x = x_raw - 1;
    c_y = y_raw - 1;
    (default) -> (junction 163)
    (junction 163) -> (junction 164) [order 1] : [(theta <= 270+ERRVAL) && (theta >= 270 - ERRVAL)]//NORTH
    (junction 163) -> (junction 165) [order 2]
    (junction 164) -> (junction 178) : {heading = NORTH;}
    (junction 165) -> (junction 166) [order 1] : [(theta <= 90+ERRVAL) && (theta >= 90-ERRVAL)]//SOUTH
    (junction 165) -> (junction 167) [order 2]
    (junction 166) -> (junction 177) : {heading = SOUTH;}
    (junction 167) -> (junction 168) [order 1] : [(theta <= 0+ERRVAL) || (theta >= 360-ERRVAL)]//EAST
    (junction 167) -> (junction 169) [order 2]
    (junction 168) -> (junction 176) : {heading = EAST;}
    (junction 169) -> (junction 170) [order 1] : [(theta <= 180+ERRVAL) && (theta >= 180-ERRVAL)]//WEST
    (junction 169) -> (junction 171) [order 2] : {heading = NONE;}
    (junction 170) -> (junction 175) : {heading = WEST;}
    (junction 171) -> (junction 172) [order 2] : [Vr == Vl]
    (junction 172) -> (junction 174) : {wrongHeading_BOOL = true;}
    (junction 171) -> (junction 173) [order 1]
    (junction 174) -> (junction 173)
    (junction 175) -> (junction 174) : {wrongHeading_BOOL = false;}
    (junction 176) -> (junction 175)
    (junction 177) -> (junction 176)
    (junction 178) -> (junction 177)
    (junction 173) -> (junction 179)
  state CalcHeading
    entry:
    y_out = y_raw;
    x_out = x_raw;
    c_x = x_raw - 1; // X and Y in C arrays are flipped
    c_y = y_raw - 1;
    during:
    y_out = y_raw;
    x_out = x_raw;
    c_x = x_raw - 1; // X and Y in C arrays are flipped
    c_y = y_raw - 1;
    (default) -> (junction 66)
    (junction 66) -> (junction 67) [order 1] : [(theta <= 270+ERRVAL) && (theta >= 270 - ERRVAL)]//NORTH
    (junction 66) -> (junction 68) [order 2]
    (junction 67) -> (junction 75) : {heading = NORTH;}
    (junction 68) -> (junction 69) [order 1] : [(theta <= 90+ERRVAL) && (theta >= 90-ERRVAL)]//SOUTH
    (junction 68) -> (junction 70) [order 2]
    (junction 69) -> (junction 74) : {heading = SOUTH;}
    (junction 70) -> (junction 71) [order 1] : [(theta <= 0+ERRVAL) || (theta >= 360-ERRVAL)]//EAST
    (junction 70) -> (junction 80) [order 2]
    (junction 71) -> (junction 73) : {heading = EAST;}
    (junction 80) -> (junction 79) [order 1] : [(theta <= 180+ERRVAL) && (theta >= 180-ERRVAL)]//WEST
    (junction 80) -> (junction 128) [order 2] : {heading = NONE;}
    (junction 79) -> (junction 77) : {heading = WEST;}
    (junction 128) -> (junction 125) [order 2] : [Vr == Vl]
    (junction 125) -> (junction 126) : {wrongHeading_BOOL = true;}
    (junction 128) -> (junction 72) [order 1]
    (junction 126) -> (junction 72)
    (junction 77) -> (junction 126) : {wrongHeading_BOOL = false;}
    (junction 73) -> (junction 77)
    (junction 74) -> (junction 73)
    (junction 75) -> (junction 74)
    (junction 72) -> (junction 76)
  (default) -> noHit
  (junction 157) -> (junction 147) [order 3] : [(heading == NORTH) ...
      | && ((c_y - 1) >= 0)...
      | &&((c_x) >= 0)]
  (junction 147) -> noHit : [room[c_y - 1][c_x] == 255]
  (junction 146) -> noHit : [room[c_y][c_x + 1] == 255]
  (junction 157) -> (junction 146) [order 2] : [(heading == EAST) ...
      | && ((c_x) <= 150 - 1)...
      | && ((c_y) >= 0)]
  (junction 92) -> HitCalcHeading : [room[c_y - 1][c_x] == 0]
  (junction 109) -> (junction 92) [order 2] : [(heading == NORTH) ...
      | && ((c_y - 1) >= 0)...
      | &&((c_x) >= 0)]
  CalcHeading -> CalcHeading [order 3] : [hasChanged(theta)]
  HitCalcHeading -> (junction 157) [order 1] : [(Vr > 0) && (Vl > 0)]//FORWARD
  (junction 157) -> (junction 148) [order 4] : [(heading == SOUTH) ...
      | && ((c_y + 1) <= 150 - 1)...
      | && ((c_x) >= 0)]
  (junction 157) -> (junction 145) [order 1] : [(heading == WEST) ...
      | && ((c_x - 1) >= 0)...
      | && ((c_y) >= 0)]
  (junction 148) -> noHit : [room[c_y + 1][c_x] == 255]
  (junction 97) -> HitCalcHeading : [room[c_y][c_x + 1] == 0]
  (junction 109) -> (junction 97) [order 4] : [(heading == EAST) ...
      | && ((c_x) <= 150 - 1)...
      | && ((c_y) >= 0)]
  CalcHeading -> (junction 109) [order 1] : [(Vr > 0) && (Vl > 0)]//FORWARD
  (junction 109) -> (junction 100) [order 1] : [(heading == SOUTH) ...
      | && ((c_y + 1) <= 150 - 1)...
      | && ((c_x) >= 0)]
  (junction 109) -> (junction 103) [order 3] : [(heading == WEST) ...
      | && ((c_x - 1) >= 0)...
      | && ((c_y) >= 0)]
  (junction 145) -> noHit : [room[c_y][c_x - 1] == 255]
  (junction 100) -> HitCalcHeading : [room[c_y + 1][c_x] == 0]
  (junction 103) -> HitCalcHeading : [room[c_y][c_x - 1] == 0]
  (junction 135) -> noHit : [room[c_y + 1][c_x] == 255]
  (junction 160) -> (junction 135) [order 1] : [(heading == NORTH) ...
      | && ((c_y + 1) <= 150 - 1)...
      | && ((c_x) >= 0)]
  (junction 111) -> (junction 113) [order 1] : [(heading == NORTH) ...
      | && ((c_y + 1) <= 150 - 1)...
      | && ((c_x) >= 0)]
  (junction 113) -> HitCalcHeading : [room[c_y + 1][c_x] == 0]
  CalcHeading -> (junction 111) [order 2] : [(Vr < 0) && (Vl < 0)]//BACKWARD
  (junction 111) -> (junction 114) [order 2] : [(heading == EAST) ...
      | && ((c_x - 1) >= 0)...
      | && ((c_y) >= 0)]
  (junction 111) -> (junction 115) [order 3] : [(heading == SOUTH) ...
      | && ((c_y - 1) >= 0)...
      | && ((c_x) >=0)]
  (junction 111) -> (junction 116) [order 4] : [(heading == WEST) ...
      | && ((c_x + 1) <= (150-1))...
      | && ((c_y) >= 0)]
  (junction 114) -> HitCalcHeading : [room[c_y][c_x - 1] == 0]
  HitCalcHeading -> (junction 160) [order 2] : [(Vr < 0) && (Vl < 0)]//BACKWARD
  (junction 160) -> (junction 138) [order 2] : [(heading == EAST) ...
      | && ((c_x - 1) >= 0)...
      | && ((c_y) >= 0)]
  (junction 138) -> noHit : [room[c_y][c_x - 1] == 255]
  (junction 160) -> (junction 134) [order 3] : [(heading == SOUTH) ...
      | && ((c_y - 1) >= 0)...
      | && ((c_x) >=0)]
  (junction 160) -> (junction 136) [order 4] : [(heading == WEST) ...
      | && ((c_x + 1) <= (150-1))...
      | && ((c_y) >= 0)]
  noHit -> CalcHeading
  (junction 115) -> HitCalcHeading : [(room[c_y - 1][c_x] == 0)]
  (junction 134) -> noHit : [room[c_y - 1][c_x] == 255]
  (junction 116) -> HitCalcHeading : [room[c_y][c_x + 1] == 0]
  (junction 136) -> noHit : [room[c_y][c_x + 1] == 255]
  data: x_raw input; y_raw input; room input size=[roomSize roomSize]; y_out output int32; x_out output int32; y_temp local int32; x_temp local int32; hit_BOOL output boolean; theta input; ERRVAL input; NORTH input; SOUTH input; EAST input; WEST input; NONE input; heading local int16; Vr input; Vl input; wrongHeading_BOOL output boolean; c_x local double; c_y local double

== stateflow chart AreaCoverageTestHarness/Robot/RoomFilterSystem/StepCalc/Chart ==
  state inStep
    entry:
    temp = 0;
    state wait
    (default) -> wait
    (junction 7) -> wait : [oldPos < pos]/temp++;
    wait -> (junction 5) [order 1] : [hasChanged(pos)]
    (junction 5) -> wait : [oldPos > pos]/temp--;
    wait -> (junction 7) [order 2] : [hasChanged(pos)]
  state IncrementStep
    entry:
    step++;
  state Start
    entry:
    step = pos;
  state decrementStep
    step--;
  (default) -> Start
  Start -> inStep
  inStep -> IncrementStep [order 1] : [temp >= STEP_SIZE]
  IncrementStep -> inStep
  decrementStep -> inStep
  inStep -> decrementStep [order 2] : [temp <= -STEP_SIZE]
  data: pos input; oldPos input; step output int32; temp local int8; STEP_SIZE input int8

== stateflow chart AreaCoverageTestHarness/Robot/OrientationCalculator/VelocityCalculator/Chart ==
  (default) -> (junction 96)
  (junction 96) -> (junction 110) [order 1] : [(!LeftMotorPosPin_BOOL && !LeftMotorNegPin_BOOL && !RightMotorPosPin_BOOL && !RightMotorNegPin_BOOL)...
      | || (LeftMotorPosPin_BOOL && LeftMotorNegPin_BOOL && !RightMotorPosPin_BOOL && !RightMotorNegPin_BOOL)...
      | || (!LeftMotorPosPin_BOOL && !LeftMotorNegPin_BOOL && RightMotorPosPin_BOOL && RightMotorNegPin_BOOL)...
      | || (LeftMotorPosPin_BOOL && LeftMotorNegPin_BOOL && RightMotorPosPin_BOOL && RightMotorNegPin_BOOL)]
  (junction 110) -> (junction 118) : {Vr  = 0;
      | Vl = 0;}
  (junction 96) -> (junction 100) [order 2]
  (junction 100) -> (junction 97) [order 1] : [(!LeftMotorPosPin_BOOL && !LeftMotorNegPin_BOOL && RightMotorPosPin_BOOL && !RightMotorNegPin_BOOL)...
      | || (!LeftMotorPosPin_BOOL && LeftMotorNegPin_BOOL && RightMotorPosPin_BOOL && RightMotorNegPin_BOOL)...
      | || (LeftMotorPosPin_BOOL && LeftMotorNegPin_BOOL && RightMotorPosPin_BOOL && !RightMotorNegPin_BOOL)...
      | || (!LeftMotorPosPin_BOOL && LeftMotorNegPin_BOOL && !RightMotorPosPin_BOOL && !RightMotorNegPin_BOOL)]
  (junction 97) -> (junction 122) : {Vr = MAX_SPEED;
      | Vl = 0;}
  (junction 100) -> (junction 99) [order 2]
  (junction 99) -> (junction 98) [order 1] : [(!LeftMotorPosPin_BOOL && !LeftMotorNegPin_BOOL && !RightMotorPosPin_BOOL && RightMotorNegPin_BOOL)...
      | || (LeftMotorPosPin_BOOL && !LeftMotorNegPin_BOOL && !RightMotorPosPin_BOOL && !RightMotorNegPin_BOOL)...
      | || (LeftMotorPosPin_BOOL && !LeftMotorNegPin_BOOL && RightMotorPosPin_BOOL && RightMotorNegPin_BOOL)...
      | || (LeftMotorPosPin_BOOL && LeftMotorNegPin_BOOL && !RightMotorPosPin_BOOL && RightMotorNegPin_BOOL)]
  (junction 98) -> (junction 86) : {Vr = 0;
      | Vl = MAX_SPEED;}
  (junction 99) -> (junction 87) [order 2]
  (junction 87) -> (junction 101) [order 1] : [(!LeftMotorPosPin_BOOL && LeftMotorNegPin_BOOL && RightMotorPosPin_BOOL && !RightMotorNegPin_BOOL)]
  (junction 87) -> (junction 102) [order 2]
  (junction 101) -> (junction 130) : {Vr = MAX_SPEED;
      | Vl = -MAX_SPEED;}
  (junction 102) -> (junction 104) [order 1] : [(LeftMotorPosPin_BOOL && !LeftMotorNegPin_BOOL && !RightMotorPosPin_BOOL && RightMotorNegPin_BOOL)]
  (junction 102) -> (junction 133) [order 2]
  (junction 104) -> (junction 88) : {Vr = -MAX_SPEED;
      | Vl = MAX_SPEED;}
  (junction 133) -> (junction 105) [order 1] : [(LeftMotorPosPin_BOOL && !LeftMotorNegPin_BOOL && RightMotorPosPin_BOOL && !RightMotorNegPin_BOOL)]
  (junction 133) -> (junction 90) [order 2]
  (junction 105) -> (junction 89) : {Vr = MAX_SPEED;
      | Vl = MAX_SPEED;}
  (junction 90) -> (junction 94) [order 1] : [(!LeftMotorPosPin_BOOL && LeftMotorNegPin_BOOL && !RightMotorPosPin_BOOL && RightMotorNegPin_BOOL)]
  (junction 90) -> (junction 91) [order 2]
  (junction 94) -> (junction 127) : {Vr = -MAX_SPEED;
      | Vl = -MAX_SPEED;}
  (junction 127) -> (junction 91)
  (junction 89) -> (junction 127)
  (junction 88) -> (junction 89)
  (junction 130) -> (junction 88)
  (junction 86) -> (junction 130)
  (junction 122) -> (junction 86)
  (junction 118) -> (junction 122)
  (junction 91) -> (junction 119)
  data: LeftMotorPosPin_BOOL input; LeftMotorNegPin_BOOL input; RightMotorPosPin_BOOL input; RightMotorNegPin_BOOL input; Vr output int16; Vl output int16; MAX_SPEED input int16

== stateflow chart AreaCoverageTestHarness/Robot/RoomFilterSystem/StepCalc1/Chart ==
  state inStep
    entry:
    temp = 0;
    state wait
    (default) -> wait
    (junction 7) -> wait : [oldPos < pos]/temp++;
    wait -> (junction 5) [order 1] : [hasChanged(pos)]
    (junction 5) -> wait : [oldPos > pos]/temp--;
    wait -> (junction 7) [order 2] : [hasChanged(pos)]
  state IncrementStep
    entry:
    step++;
  state Start
    entry:
    step = pos;
  state decrementStep
    step--;
  (default) -> Start
  Start -> inStep
  inStep -> IncrementStep [order 1] : [temp >= STEP_SIZE]
  IncrementStep -> inStep
  decrementStep -> inStep
  inStep -> decrementStep [order 2] : [temp <= -STEP_SIZE]
  data: pos input; oldPos input; step output int32; temp local int8; STEP_SIZE input int8
